simulink model "step_simulink_NL_val"  (R2015b)
settings: Solver=FixedStepAuto  StartTime=0.0  StopTime=10.22  FixedStep=0.02  RelTol=1e-3
settings Model: Creator=guilh_000  LastModifiedBy=guilh_000

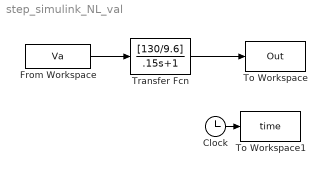
== system step_simulink_NL_val ==
  Clock : Clock
  From Workspace : FromWorkspace  VariableName=Va  SampleTime=0
  To Workspace : ToWorkspace  VariableName=Out  SampleTime=-1
  To Workspace1 : ToWorkspace  VariableName=time  SampleTime=-1
  Transfer Fcn : TransferFcn  Numerator=[130/9.6]  Denominator=[.15 1]
  wires:
  From Workspace/1 -> Transfer Fcn/1
  Transfer Fcn/1 -> To Workspace/1
  Clock/1 -> To Workspace1/1
